simulink model "impedanceSimulink"  (R2025b)
settings: Solver=VariableStepAuto  StartTime=0.0  StopTime=10.0  RelTol=1e-3
settings Model: Creator=jayde  LastModifiedBy=jayde

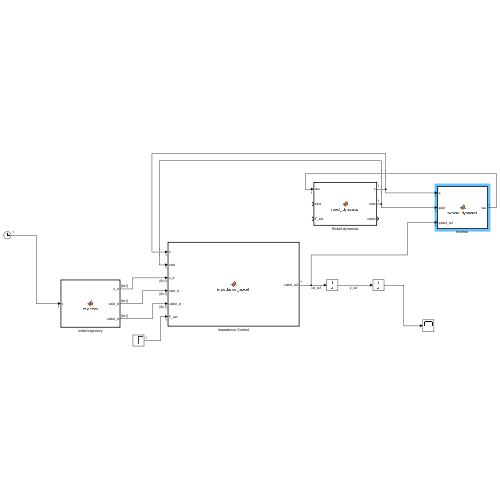
[thumbnail: Simulink's stored preview of the top-level diagram]
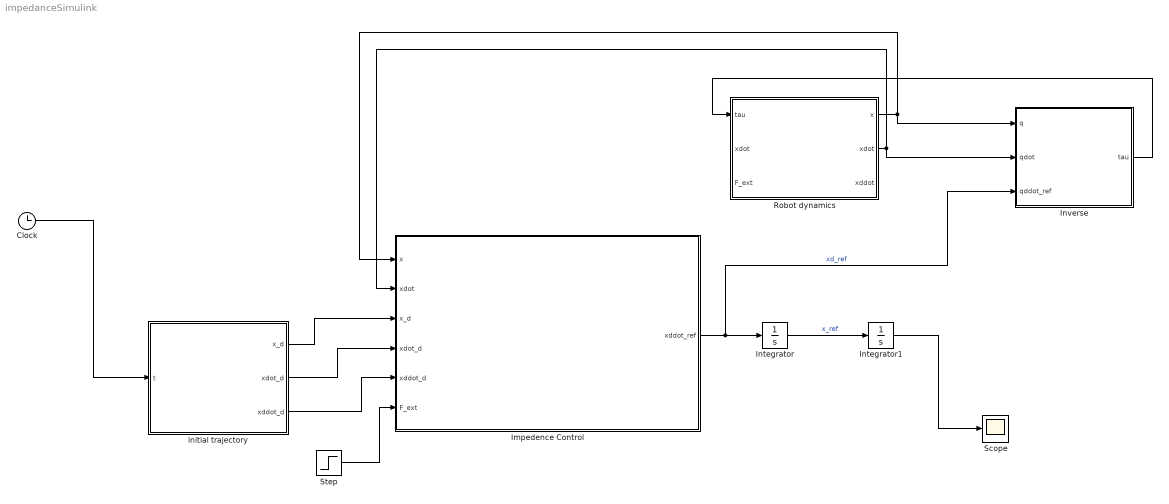
== system impedanceSimulink ==
  Clock : Clock
  Impedence Control : MATLAB Function  TreatAsAtomicUnit=on
  Integrator : Integrator
  Integrator1 : Integrator
  "Inverse " : MATLAB Function  TreatAsAtomicUnit=on
  Robot dynamics : MATLAB Function  TreatAsAtomicUnit=on
  Scope : Scope
  Step : Step  Time=5  SampleTime=0
  initial trajectory : MATLAB Function  TreatAsAtomicUnit=on
  wires:
  Clock/1 -> initial trajectory/1(t)
  Integrator/1 -> Integrator1/1  "x_ref"
  Impedence Control/1(xddot_ref) -> "Inverse "/3(qddot_ref), Integrator/1  "xd_ref"
  initial trajectory/1(x_d) -> Impedence Control/3(x_d)
  initial trajectory/2(xdot_d) -> Impedence Control/4(xdot_d)
  initial trajectory/3(xddot_d) -> Impedence Control/5(xddot_d)
  Robot dynamics/1(x) -> "Inverse "/1(q), Impedence Control/1(x)
  Robot dynamics/2(xdot) -> "Inverse "/2(qdot), Impedence Control/2(xdot)
  "Inverse "/1(tau) -> Robot dynamics/1(tau)
  Step/1 -> Impedence Control/6(F_ext)
  Integrator1/1 -> Scope/1

== matlab function impedanceSimulink/Robot dynamics ==
  data: x output; xdot output; xddot output; tau input; xdot input; F_ext input
function [x, xdot, xddot] = robot_dynamics(tau, xdot, F_ext)

persistent robot

if isempty(robot)
    robot = loadrobot("kinovaGen3", "DataFormat","column");
    robot.Gravity = [0 0 -9.81];
end

M = eye(3);
C = zeros(3);
G = [0;0;9.81];
J = eye(3);

xddot = M \ (tau + J'*F_ext - C*xdot - G);

end

== matlab function impedanceSimulink/Impedence Control ==
  data: x input; xdot input; x_d input; xdot_d input; xddot_d input; F_ext input; xddot_ref output
function xddot_ref  = impedance_model(x, xdot, x_d, xdot_d, xddot_d, F_ext)

Md = diag([1,1,1]);
Bd = diag([20,20,20]);
Kd = diag([50,50,50]);

e = x - x_d;
edot = xdot - xdot_d;

xddot_ref = xddot_d + Md \ (F_ext - Bd.*edot - Kd*e);

end

== matlab function impedanceSimulink/Inverse  ==
  data: q input; tau output; qdot input; qddot_ref input
function tau = inverse_dynamics(q, qdot, qddot_ref)

robot = rigidBodyTree;
M = massMatrix(robot, q);
C = velocityProduct(robot, q, qdot);
G = gravityTorque(robot, q);

tau = M.*qddot_ref + C.*qdot + G;

end

== matlab function impedanceSimulink/initial trajectory ==
  data: t input; x_d output; xdot_d output; xddot_d output
function [x_d, xdot_d, xddot_d] = trajectory(t)

x_d = zeros(6,1);
xdot_d = zeros(6,1);
xddot_d = zeros(6,1); 

end
